simulink model "rate_adaptive_test_module"  (R2017b)
settings: Solver=FixedStepAuto  StartTime=0.0  StopTime=120  FixedStep=0.001  RelTol=1e-3  EnableMultiTasking=on
libraries: frdmk64flib x1, dspstat3 x1
settings Model: ExtModeTrigDuration=5  Creator=puerstee  LastModifiedBy=puerstee
settings OptimizationCC: PassReuseOutputArgsAs=Individual arguments  MaxStackSize=64
settings DebuggingCC: ParameterTunabilityLossMsg=error
settings HardwareCC: ProdBitPerPointer=32  ProdBitPerSizeT=32  ProdBitPerPtrDiffT=32  ProdLargestAtomicInteger=Long  ProdLargestAtomicFloat=Double  ProdWordSize=32  ProdHWDeviceType=ARM Compatible->ARM Cortex
settings SFSimCC: MATLABDynamicMemAlloc=off
settings RTWCC: SystemTargetFile=ert.tlc  HardwareBoard=NXP FRDM-K64F  TemplateMakefile=ert_default_tmf  GenerateReport=on  Toolchain=GNU Tools for ARM Embedded Processors  IncludeHyperlinkInReport=on  LaunchReport=on  GenerateTraceInfo=on  GenerateTraceReport=on  GenerateTraceReportSl=on  GenerateTraceReportSf=on  GenerateTraceReportEml=on
settings CodeAppCC: ForceParamTrailComments=on  IgnoreCustomStorageClasses=off  OperatorAnnotations=on  SimulinkDataObjDesc=on  SFDataObjDesc=on  InsertBlockDesc=on

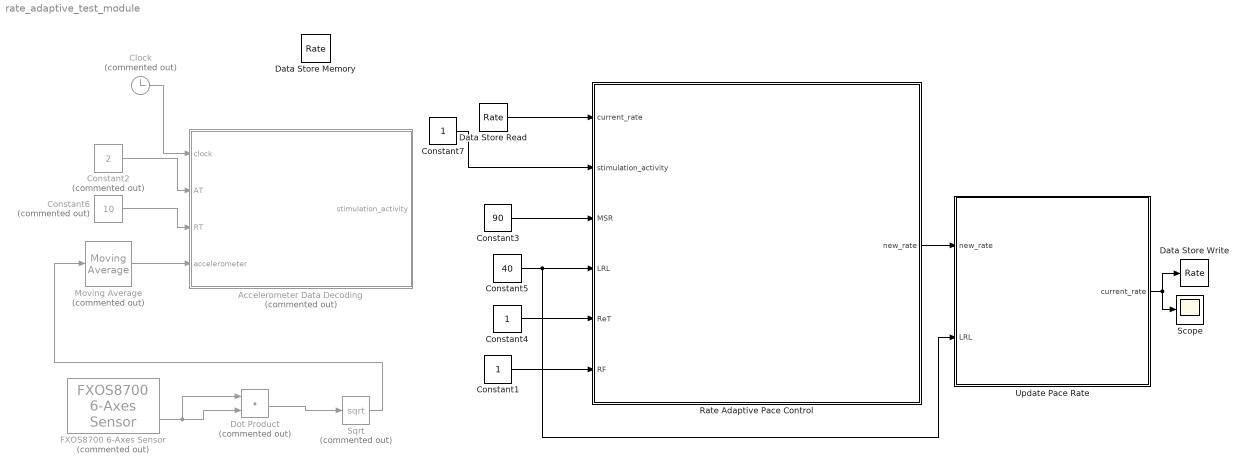
== system rate_adaptive_test_module ==
  "Accelerometer Data Decoding " : Stateflow chart  Commented=on  TreatAsAtomicUnit=on
  Clock : Clock  Commented=on
  Constant1 : Constant  OutDataTypeStr=single
  Constant2 : Constant  Commented=on  Value=2  OutDataTypeStr=int16
  Constant3 : Constant  Value=90  OutDataTypeStr=single
  Constant4 : Constant  OutDataTypeStr=single
  Constant5 : Constant  Value=40  OutDataTypeStr=single
  Constant6 : Constant  Commented=on  Value=10  OutDataTypeStr=int16
  Constant7 : Constant  OutDataTypeStr=boolean
  Data Store Memory : DataStoreMemory  DataStoreName=Rate  ReadBeforeWriteMsg=warning  WriteAfterWriteMsg=warning  WriteAfterReadMsg=warning  ShowAdditionalParam=off  OutDataTypeStr=single
  Data Store Read : DataStoreRead  DataStoreName=Rate  DataStoreElements=Rate
  Data Store Write : DataStoreWrite  DataStoreName=Rate  DataStoreElements=Rate
  Dot Product : DotProduct  Commented=on  InputSameDT=on  OutDataTypeStr=Inherit: Inherit via internal rule
  FXOS8700 6-Axes Sensor : frdmk64flib/FXOS8700 6-Axes Sensor  Commented=on  Activesensor=Accelerometer and Magnetometer  ODR=800Hz  HybridODR=400Hz  Accelfullrange=-4g to +4g  SampleTime=-1
      settings: SourceProductName=Simulink Coder Support Package for NXP FRDM-K64F Board
  Moving Average : dspstat3/Moving Average  Commented=on  Method=Sliding window  SpecifyWindowLength=on  WindowLength=500  ForgettingFactor=0.9  SimulateUsing=Code generation
  "Rate Adaptive Pace Control " : Stateflow chart  TreatAsAtomicUnit=on
  Scope : Scope
  Sqrt : Sqrt  Commented=on  SaturateOnIntegerOverflow=on
  "Update Pace Rate " : Stateflow chart  TreatAsAtomicUnit=on
  wires:
  Constant1/1 -> "Rate Adaptive Pace Control "/6(RF)
  Constant3/1 -> "Rate Adaptive Pace Control "/3(MSR)
  Constant4/1 -> "Rate Adaptive Pace Control "/5(ReT)
  Constant5/1 -> "Update Pace Rate "/2(LRL), "Rate Adaptive Pace Control "/4(LRL)
  Data Store Read/1 -> "Rate Adaptive Pace Control "/1(current_rate)
  "Update Pace Rate "/1(current_rate) -> Scope/1, Data Store Write/1
  Constant2/1 -> "Accelerometer Data Decoding "/2(AT)
  FXOS8700 6-Axes Sensor/2 -> Dot Product/1, Dot Product/2
  Dot Product/1 -> Sqrt/1
  Constant6/1 -> "Accelerometer Data Decoding "/3(RT)
  Moving Average/1 -> "Accelerometer Data Decoding "/4(accelerometer)
  Clock/1 -> "Accelerometer Data Decoding "/1(clock)
  Sqrt/1 -> Moving Average/1
  "Rate Adaptive Pace Control "/1(new_rate) -> "Update Pace Rate "/1(new_rate)
  Constant7/1 -> "Rate Adaptive Pace Control "/2(stimulation_activity)

== stateflow chart rate_adaptive_test_module/Update Pace Rate  ==
  state initialization_state
    entry: current_rate = LRL;
  state continuous_state
    entry: current_rate = new_rate;
  (default) -> initialization_state
  initialization_state -> continuous_state : [after((1000),msec)]
  continuous_state -> continuous_state : [after((1000),msec)]
  data: current_rate output single; new_rate input single; LRL input single

== stateflow chart rate_adaptive_test_module/Accelerometer Data Decoding  ==
  state False
    entry:
    stimulation_activity = false;
  state Compare_State
    entry:
    compare = clock - time;
  state True
    entry: stimulation_activity = true;
  (default) -> False
  True -> False : [accelerometer<AT]
  Compare_State -> False [order 1] : [accelerometer<AT]
  False -> Compare_State : [accelerometer>=AT]{time=clock}
  Compare_State -> Compare_State [order 2] : [compare<RT]
  Compare_State -> True [order 3] : [compare>=RT]
  data: clock input; stimulation_activity output boolean; AT input int16; RT input int16; accelerometer input double; time local; compare local

== stateflow chart rate_adaptive_test_module/Rate Adaptive Pace Control  ==
  state const_LRL
    entry: new_rate=LRL;
  state increasing_rate
  state decreasing_rate
  state const_MSR
    entry: new_rate=MSR;
  (default) -> const_LRL : {new_rate=LRL}
  decreasing_rate -> const_LRL [order 2] : [after((1000),msec) && current_rate + (LRL-MSR)/(60*ReT) <= LRL]
  const_LRL -> increasing_rate : [stimulation_activity==true]
  increasing_rate -> decreasing_rate [order 1] : [stimulation_activity==false]
  increasing_rate -> increasing_rate [order 3] : [(current_rate+ (MSR/LRL)*RF)<MSR && after((1000),msec)]
      | {new_rate=current_rate + (MSR/LRL)*RF}
  decreasing_rate -> decreasing_rate [order 3] : [after((1000),msec) && current_rate + (LRL-MSR)/(60*ReT) > LRL]
      | {new_rate=current_rate + (LRL-MSR)/(60*ReT)}
  decreasing_rate -> increasing_rate [order 1] : [stimulation_activity==true]
  const_MSR -> decreasing_rate : [stimulation_activity==false]
  increasing_rate -> const_MSR [order 2] : [(current_rate+ (MSR/LRL)*RF) >= MSR && after((1000),msec)]
  data: new_rate output single; current_rate input single; stimulation_activity input boolean; MSR input single; LRL input single; ReT input single; RF input single
